simulink model "TEST_IPM_2_0"  (R2019b)
settings: configuration reference "Configuration" (kept outside this file)
PreLoadFcn:
  | RTWConfigurationCB('preloadfcn', bdroot);
values from neighbouring files (symbols this model uses):
  MParamFbase = 200.0    [TEST_IPM_LIB.sldd]
  MParamIbase = 360.0    [TEST_IPM_LIB.sldd]
  MParamLd = 0.002    [TEST_IPM_LIB.sldd]
  MParamLq = 0.002    [TEST_IPM_LIB.sldd]
  MParamRs = 1.15    [TEST_IPM_LIB.sldd]
  PWM_TPBRD_HALF = 5000.0    [TEST_IPM_LIB.sldd]
  Ts_10kHz = 0.0001    [TEST_IPM_LIB.sldd]
  Ts_1kHz = 0.001    [TEST_IPM_LIB.sldd]
undefined symbols (not defined in the file or in its folder): Down, GPTRIP1SEL, GPTRIP2SEL, TZ1, TZ2, Up
libraries: c280xlib x66, c2837xDlib x18, c2802xlib x10, powerlib_meascontrol x9, dsparch4 x4, c2000lib x1, c2806xlib x1, idelinklib_common x1
(part 3 of 6)

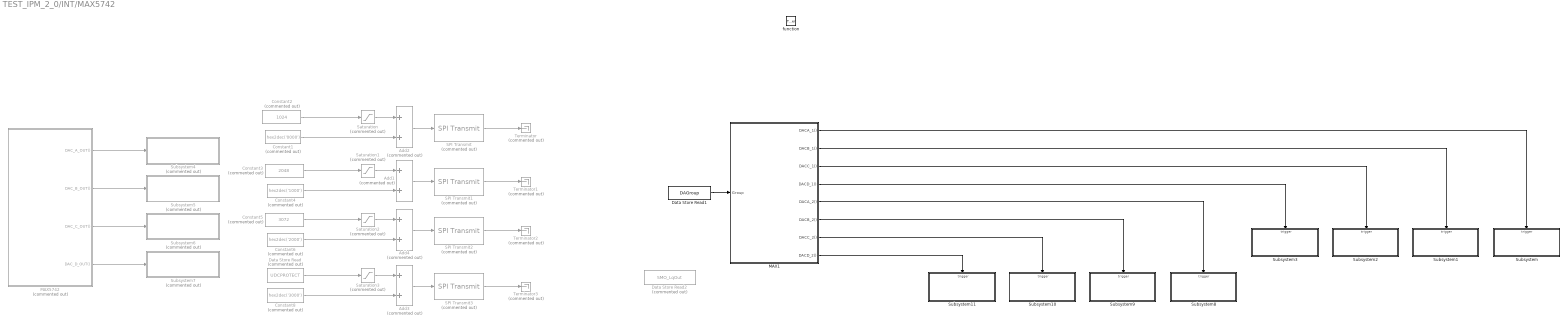
== system TEST_IPM_2_0/INT/MAX5742 ==
  function : TriggerPort  TriggerType=function-call  VariantControl=Variant
  Add{1..4} (4 alike) : Sum  Commented=on
  Constant1 : Constant  Commented=on  Value=hex2dec('0000')  OutDataTypeStr=uint16  SampleTime=-1
  Constant2 : Constant  Priority=102  Commented=on  Value=1024  OutDataTypeStr=Inherit: Inherit via back propagation  SampleTime=-1
  Constant3 : Constant  Priority=107  Commented=on  Value=2048  OutDataTypeStr=Inherit: Inherit via back propagation  SampleTime=-1
  Constant4 : Constant  Commented=on  Value=hex2dec('1000')  OutDataTypeStr=uint16  SampleTime=-1
  Constant5 : Constant  Priority=112  Commented=on  Value=3072  OutDataTypeStr=Inherit: Inherit via back propagation  SampleTime=-1
  Constant6 : Constant  Commented=on  Value=hex2dec('2000')  OutDataTypeStr=uint16  SampleTime=-1
  Constant8 : Constant  Commented=on  Value=hex2dec('3000')  OutDataTypeStr=uint16  SampleTime=-1
  Data Store Read : DataStoreRead  Commented=on  DataStoreName=UDCPROTECT
  Data Store Read1 : DataStoreRead  DataStoreName=DAGroup
  Data Store Read2 : DataStoreRead  Commented=on  DataStoreName=SMO_LqOut
  MAX1 : MATLAB Function  TreatAsAtomicUnit=on
  MAX5742 : Stateflow chart  Commented=on  BlockKeywords=__PRM__SERIALIZED__DATA__:Stateflow Chart,Stateflow Diagram  TreatAsAtomicUnit=on
  SPI Transmit : c280xlib/SPI Transmit  Commented=on  SPISelect=SPI_B  ClockPolarity=Falling_edge  ClockPhase=No_delay  SPIModule=uint32(0)  Mode=Master  BusSpeed=uint32(1000000)  FirstBitToTransfer=Most significant bit (MSB)  ClockMode=0  BlockFunction=Write  EnableRegisterAddress=on  RegisterAddress=0  OutputDataType=int8  OutputDataLength=1  BlockingMode=off  DataBits=16  UseCustomSSPin=Provided by the SPI peripheral  ActiveLowSSPin=Active low  Pin=0
      settings: SourceProductName=Embedded Coder Support Package for Texas Instruments C2000 Processors  SourceProductBaseCode=TIC2000
  SPI Transmit1 : c280xlib/SPI Transmit  Commented=on  SPISelect=SPI_B  ClockPolarity=Rising_edge  ClockPhase=No_delay  SPIModule=uint32(0)  Mode=Master  BusSpeed=uint32(1000000)  FirstBitToTransfer=Most significant bit (MSB)  ClockMode=0  BlockFunction=Write  EnableRegisterAddress=on  RegisterAddress=0  OutputDataType=int8  OutputDataLength=1  BlockingMode=off  DataBits=16  UseCustomSSPin=Provided by the SPI peripheral  ActiveLowSSPin=Active low  Pin=0
      settings: SourceProductName=Embedded Coder Support Package for Texas Instruments C2000 Processors  SourceProductBaseCode=TIC2000
  SPI Transmit2 : c280xlib/SPI Transmit  Commented=on  SPISelect=SPI_B  ClockPolarity=Rising_edge  ClockPhase=No_delay  SPIModule=uint32(0)  Mode=Master  BusSpeed=uint32(1000000)  FirstBitToTransfer=Most significant bit (MSB)  ClockMode=0  BlockFunction=Write  EnableRegisterAddress=on  RegisterAddress=0  OutputDataType=int8  OutputDataLength=1  BlockingMode=off  DataBits=16  UseCustomSSPin=Provided by the SPI peripheral  ActiveLowSSPin=Active low  Pin=0
      settings: SourceProductName=Embedded Coder Support Package for Texas Instruments C2000 Processors  SourceProductBaseCode=TIC2000
  SPI Transmit3 : c280xlib/SPI Transmit  Commented=on  SPISelect=SPI_B  ClockPolarity=Rising_edge  ClockPhase=No_delay  SPIModule=uint32(0)  Mode=Master  BusSpeed=uint32(1000000)  FirstBitToTransfer=Most significant bit (MSB)  ClockMode=0  BlockFunction=Write  EnableRegisterAddress=on  RegisterAddress=0  OutputDataType=int8  OutputDataLength=1  BlockingMode=off  DataBits=16  UseCustomSSPin=Provided by the SPI peripheral  ActiveLowSSPin=Active low  Pin=0
      settings: SourceProductName=Embedded Coder Support Package for Texas Instruments C2000 Processors  SourceProductBaseCode=TIC2000
  Saturation{,1..3} (4 alike) : Saturate  Commented=on  UpperLimit=4095  LowerLimit=0  OutDataTypeStr=uint16
  Subsystem : Subsystem
  Subsystem1 : Subsystem
  Subsystem10 : Subsystem
  Subsystem11 : Subsystem
  Subsystem2 : Subsystem
  Subsystem3 : Subsystem
  Subsystem4 : Subsystem  Commented=on
  Subsystem5 : Subsystem  Commented=on
  Subsystem6 : Subsystem  Commented=on
  Subsystem7 : Subsystem  Commented=on
  Subsystem8 : Subsystem
  Subsystem9 : Subsystem
  Terminator{,1..3} (4 alike) : Terminator  Commented=on
  wires:
  MAX1/4(DACD_1()) -> Subsystem3/Trigger
  MAX1/3(DACC_1()) -> Subsystem2/Trigger
  MAX1/2(DACB_1()) -> Subsystem1/Trigger
  MAX1/1(DACA_1()) -> Subsystem/Trigger
  SPI Transmit/1 -> Terminator/1
  Add2/1 -> SPI Transmit/1
  Saturation/1 -> Add2/1
  Constant2/1 -> Saturation/1
  Constant1/1 -> Add2/2
  SPI Transmit1/1 -> Terminator1/1
  Constant4/1 -> Add1/2
  Add1/1 -> SPI Transmit1/1
  Saturation1/1 -> Add1/1
  Constant3/1 -> Saturation1/1
  Constant5/1 -> Saturation2/1
  Constant6/1 -> Add4/2
  Add4/1 -> SPI Transmit2/1
  Saturation2/1 -> Add4/1
  SPI Transmit2/1 -> Terminator2/1
  Saturation3/1 -> Add3/1
  Add3/1 -> SPI Transmit3/1
  SPI Transmit3/1 -> Terminator3/1
  Constant8/1 -> Add3/2
  Data Store Read/1 -> Saturation3/1
  MAX5742/1(DAC_A_OUT()) -> Subsystem4/Trigger
  MAX5742/2(DAC_B_OUT()) -> Subsystem5/Trigger
  MAX5742/3(DAC_C_OUT()) -> Subsystem6/Trigger
  MAX5742/4(DAC_D_OUT()) -> Subsystem7/Trigger
  MAX1/5(DACA_2()) -> Subsystem8/Trigger
  MAX1/6(DACB_2()) -> Subsystem9/Trigger
  MAX1/7(DACC_2()) -> Subsystem10/Trigger
  MAX1/8(DACD_2()) -> Subsystem11/Trigger
  Data Store Read1/1 -> MAX1/1(Group)

== system TEST_IPM_2_0/INT/Motor Control ==
  function : TriggerPort  TriggerType=function-call  VariantControl=Variant
  Adjusting Mode : Subsystem  TreatAsAtomicUnit=on
  Clark Transformation : Subsystem
  Current_PI : Subsystem  TreatAsAtomicUnit=on
      settings: RTWSystemCode=Inline
  Data Store Read : DataStoreRead  DataStoreName=U_Current
  Data Store Read1 : DataStoreRead  DataStoreName=ControlAng
  Data Store Read2 : DataStoreRead  DataStoreName=ControlMode
  Data Store Read5 : DataStoreRead  DataStoreName=V_Current
  Data Store Read6 : DataStoreRead  DataStoreName=W_Current
  Data Store Write : DataStoreWrite  DataStoreName=COMPARE_A
  Data Store Write1 : DataStoreWrite  DataStoreName=COMPARE_B
  Data Store Write2 : DataStoreWrite  DataStoreName=COMPARE_C
  Data Store Write3 : DataStoreWrite  DataStoreName=Beta_Current
  Data Store Write4 : DataStoreWrite  DataStoreName=Alpha_Current
  Demux : Demux  Outputs=3
  Error : Subsystem  TreatAsAtomicUnit=on
  IF : Subsystem  TreatAsAtomicUnit=on
  Park Transformation : Subsystem
  SVPWM : Subsystem  TreatAsAtomicUnit=on
      settings: RTWSystemCode=Inline
  SpeedMode : Subsystem  TreatAsAtomicUnit=on
  "Stop " : Subsystem  TreatAsAtomicUnit=on
  Switch Case : SwitchCase  CaseConditions={0,1,2,3,4,5}
  TorqueMode : Subsystem  TreatAsAtomicUnit=on
  VF : Subsystem  TreatAsAtomicUnit=on
  wires:
  Data Store Read2/1 -> Switch Case/1
  Switch Case/1 -> Adjusting Mode/Action
  Switch Case/6 -> "Stop "/Action
  Switch Case/7 -> Error/Action
  Switch Case/2 -> VF/Action
  Switch Case/3 -> IF/Action
  Switch Case/4 -> TorqueMode/Action
  Switch Case/5 -> SpeedMode/Action
  Clark Transformation/2(Beta) -> Data Store Write3/1, Park Transformation/2(Beta)
  Clark Transformation/1(Alpha) -> Data Store Write4/1, Park Transformation/1(Alpha)
  Data Store Read1/1 -> SVPWM/3(Angle), Park Transformation/3(theta)
  Data Store Read/1 -> Clark Transformation/1(U)
  Data Store Read5/1 -> Clark Transformation/2(V)
  Data Store Read6/1 -> Clark Transformation/3(W)
  Park Transformation/1(D) -> Current_PI/1(Id_FeedBack)
  Park Transformation/2(Q) -> Current_PI/2(Iq_FeedBack)
  Current_PI/1(Ud_Reference) -> SVPWM/1(Ud_Reference)
  Current_PI/2(Uq_Reference) -> SVPWM/2(Uq_Reference)
  SVPWM/1(COMPARE) -> Demux/1
  Demux/1 -> Data Store Write/1
  Demux/2 -> Data Store Write1/1
  Demux/3 -> Data Store Write2/1

== system TEST_IPM_2_0/INT/Read Rotor Position ==
  function : TriggerPort  TriggerType=function-call  VariantControl=Variant
  Add : Sum  Inputs=+-  OutDataTypeStr=int16
  Constant1 : Constant  Value=10000  OutDataTypeStr=int16  SampleTime=-1
  Constant2 : Constant  Value=2*pi  OutDataTypeStr=single  SampleTime=-1
  Data Store Read : DataStoreRead  Priority=3  Commented=on  DataStoreName=SPIC_Tx
  Data Store Read1 : DataStoreRead  Priority=5  Commented=on  DataStoreName=SPIC_Tx
  Data Store Read2 : DataStoreRead  DataStoreName=QEP_OFFSET
  Data Store Read3 : DataStoreRead  Commented=on  DataStoreName=ResloverMid
  Data Store Write : DataStoreWrite  Commented=on  DataStoreName=ResloverAng
  Data Store Write1 : DataStoreWrite  Commented=on  DataStoreName=SPIC_Rx
  Data Store Write2 : DataStoreWrite  Commented=on  DataStoreName=N_FBK
  Data Store Write3 : DataStoreWrite  Commented=on  DataStoreName=ResloverFaultRead
  Data Store Write4 : DataStoreWrite  DataStoreName=QEP_RAW
  Data Store Write5 : DataStoreWrite  DataStoreName=ResloverAng
  Data Store Write6 : DataStoreWrite  DataStoreName=QEP_ANGLE
  Data Store Write7 : DataStoreWrite  DataStoreName=N_FBK
  Digital Output1 : c2837xDlib/Digital Output  Commented=on  GPIO_Number=GPIO48~GPIO55  GPIO_Bit0=off  GPIO_BIT0_Toggle=off  GPIO_Bit1=off  GPIO_BIT1_Toggle=off  GPIO_Bit2=off  GPIO_BIT2_Toggle=off  GPIO_Bit3=off  GPIO_BIT3_Toggle=off  GPIO_Bit4=off  GPIO_BIT4_Toggle=off  GPIO_Bit5=on  GPIO_BIT5_Toggle=off  GPIO_Bit6=off  GPIO_BIT6_Toggle=off  GPIO_Bit7=off  GPIO_BIT7_Toggle=off
      settings: SourceProductName=Embedded Coder Support Package for Texas Instruments C2000 Processors  SourceProductBaseCode=TIC2000
  Digital Output2 : c2837xDlib/Digital Output  Commented=on  GPIO_Number=GPIO48~GPIO55  GPIO_Bit0=off  GPIO_BIT0_Toggle=off  GPIO_Bit1=off  GPIO_BIT1_Toggle=off  GPIO_Bit2=off  GPIO_BIT2_Toggle=off  GPIO_Bit3=off  GPIO_BIT3_Toggle=off  GPIO_Bit4=off  GPIO_BIT4_Toggle=off  GPIO_Bit5=off  GPIO_BIT5_Toggle=off  GPIO_Bit6=on  GPIO_BIT6_Toggle=off  GPIO_Bit7=off  GPIO_BIT7_Toggle=off
      settings: SourceProductName=Embedded Coder Support Package for Texas Instruments C2000 Processors  SourceProductBaseCode=TIC2000
  Gain : Gain  Commented=on  Gain=2*pi
  Gain1 : Gain  Gain=5  OutDataTypeStr=single
  Gain2 : Gain  Gain=2*pi/10000  OutDataTypeStr=single
  MATLAB Function : MATLAB Function  Commented=on  TreatAsAtomicUnit=on
  MATLAB Function1 : MATLAB Function  TreatAsAtomicUnit=on
  Mod : Math  Operator=mod  SignedPower=off  OutputSignalType=real  SaturateOnIntegerOverflow=on
  Mod1 : Math  Operator=mod  SignedPower=off  OutputSignalType=real  SaturateOnIntegerOverflow=on
  "RAW_DATA2Angle " : MATLAB Function  Commented=on  TreatAsAtomicUnit=on
  ResloverWR1 : Constant  Priority=6  Commented=on  OutDataTypeStr=Inherit: Inherit via back propagation  SampleTime=-1
  ResloverWR2 : Constant  Priority=6  Commented=on  OutDataTypeStr=Inherit: Inherit via back propagation  SampleTime=-1
  SPI Master Transfer : c280xlib/SPI Master Transfer  Commented=on  SPISelect=SPI_C  ClockPolarity=Rising_edge  ClockPhase=No_delay  SPIModule=uint32(0)  Mode=Master  BusSpeed=uint32(1000000)  FirstBitToTransfer=Most significant bit (MSB)  ClockMode=0  BlockFunction=Transfer  EnableRegisterAddress=off  RegisterAddress=0  OutputDataType=int8  OutputDataLength=1  DataBits=16  UseCustomSSPin=Provided by the SPI peripheral  ActiveLowSSPin=Active low  Pin=1
      settings: SourceProductName=Embedded Coder Support Package for Texas Instruments C2000 Processors  SourceProductBaseCode=TIC2000
  SPI Master Transfer1 : c280xlib/SPI Master Transfer  Commented=on  SPISelect=SPI_C  ClockPolarity=Rising_edge  ClockPhase=No_delay  SPIModule=uint32(0)  Mode=Master  BusSpeed=uint32(1000000)  FirstBitToTransfer=Most significant bit (MSB)  ClockMode=0  BlockFunction=Transfer  EnableRegisterAddress=off  RegisterAddress=0  OutputDataType=int8  OutputDataLength=1  DataBits=8  UseCustomSSPin=Provided by the SPI peripheral  ActiveLowSSPin=Active low  Pin=1
      settings: SourceProductName=Embedded Coder Support Package for Texas Instruments C2000 Processors  SourceProductBaseCode=TIC2000
  SpeedCal : Subsystem  Commented=on  TreatAsAtomicUnit=on
  SpeedCal1 : Subsystem  TreatAsAtomicUnit=on
  eQEP : c280xlib/eQEP  useModule=eQEP2  pcInputmode=Quadrature-count  externalClockrate=2x resolution: Count the rising/falling edge  swapPolarityselection=Clockwise  qdfOutputport=off  qapPolarityselection=off  qbpPolarityselection=off  qipPolarityselection=off  qspPolarityselection=off  igatePolarityselection=off  sampleTime=-1  pcOutputport=on  pcMaximumvalue=10000  indexInitializationcheck=off  indexInitializationevent=Rising edge  strobeInitializationcheck=off  strobeInitializationevent=Rising edge  softwareInitializationcheck=off  softwareInitializationsource=Set to init value at start up  softwareInitializationmode=on  pcInitialvalue=2147483648  pcResetmode=Reset on an index event  ieloutputport=off  indexEventlatch=Rising edge  seloutputport=off  strobeEventlatch=Rising edge  pcefOutputport=off  enableEqepcapture=off  qctmrOutputport=off  qcprdOutputport=off  captureTimerprescaler=128  upEventprescaler=128  overflowErrorflag=off  directionErrorflag=off  captureTimerposition=On position counter read  unitTimerperiod=100000000  captureTimerlatch=off  capturePeriodlatch=off  positionCounterlatch=off  soenPolarityselection=off  spselPolarityselection=Index pin is used for sync output  compareValuesource=Specify via dialog  shadowMode=Load on QPOSCNT=0  compareValue=4294967295  syncOutputwidth=1  polaritySyncoutput=Active high  watchdogEnable=off  watchdogTimer=65535  outport1Datatype=auto  outport2Datatype=auto  outport3Datatype=auto  outport4Datatype=auto  outport5Datatype=auto  outport6Datatype=auto  outport7Datatype=auto  outport8Datatype=auto  outport9Datatype=auto  outport10Datatype=auto  outport11Datatype=auto  outport12Datatype=auto  eqepinterrupt_pce=off  eqepinterrupt_qpe=off  eqepinterrupt_qdc=off  eqepinterrupt_wto=off  eqepinterrupt_pcu=off  eqepinterrupt_pco=off  eqepinterrupt_pcr=off  eqepinterrupt_pcm=off  eqepinterrupt_sel=off  eqepinterrupt_iel=off  eqepinterrupt_uto=off  pheOutputport=off  watchdogOutputport=off  outport13Datatype=auto  outport14Datatype=auto
      settings: SourceProductName=Embedded Coder Support Package for Texas Instruments C2000 Processors  SourceProductBaseCode=TIC2000
  wires:
  Data Store Read/1 -> SPI Master Transfer/1
  SPI Master Transfer/1 -> Data Store Write1/1, "RAW_DATA2Angle "/1(Raw_Data)
  ResloverWR1/1 -> Digital Output1/1
  Data Store Read3/1 -> "RAW_DATA2Angle "/2(Mid_Position)
  "RAW_DATA2Angle "/1(Angle_out) -> Gain/1
  SpeedCal/1(Out1) -> Data Store Write2/1
  MATLAB Function/1(FunCall()) -> SpeedCal/Trigger
  Data Store Read1/1 -> SPI Master Transfer1/1
  SPI Master Transfer1/1 -> Data Store Write3/1
  ResloverWR2/1 -> Digital Output2/1
  Gain/1 -> SpeedCal/1(In1), Data Store Write/1
  eQEP/1 -> Data Store Write4/1, Add/1
  Data Store Read2/1 -> Add/2
  Add/1 -> Mod/1
  Mod/1 -> Gain2/1
  Constant1/1 -> Mod/2
  Gain2/1 -> Gain1/1, SpeedCal1/1(In1), Data Store Write6/1
  Mod1/1 -> Data Store Write5/1
  Gain1/1 -> Mod1/1
  Constant2/1 -> Mod1/2
  MATLAB Function1/1(FunCall()) -> SpeedCal1/Trigger
  SpeedCal1/1(Out1) -> Data Store Write7/1

== system TEST_IPM_2_0/INT/ePWM ==
  function : TriggerPort  TriggerType=function-call  VariantControl=Variant
  Constant2 : Constant  Value=[0 0]  OutDataTypeStr=uint16  SampleTime=-1
  Constant3 : Constant  Value=[1 2]  OutDataTypeStr=uint16  SampleTime=-1
  Data Store Read1 : DataStoreRead  DataStoreName=STOP
  Data Store Read3 : DataStoreRead  DataStoreName=COMPARE_A
  Data Store Read4 : DataStoreRead  DataStoreName=COMPARE_B
  Data Store Read7 : DataStoreRead  DataStoreName=COMPARE_C
  Demux : Demux  Outputs=2
  If : If  IfExpression=u1 == 1
  If Action Subsystem : Subsystem  TreatAsAtomicUnit=on
  Switch : Switch  Criteria=u2 ~= 0
  ePWM : c2802xlib/ePWM  useModule=ePWM1  ePWMxLINKTBPRD=Not Linked  periodUnits=Clock cycles  timerSource=Specify via dialog  timerPeriod_clk=PWM_TPBRD  timerPeriod_sec=Tsw  tbshadow=Counter equals to zero  countingMode=Up-Down  phaseActiveEnable=Disable  phaseDirection=Count down after sync  phaseActive=0  synchronizationEnable=off  dcaevt1Sync=off  dcbevt1Sync=off  synchronizationOption=Counter equals to zero (CTR=Zero)  clockPrescale=1  HSclockPrescale=1  enswap=off  ePWMxAStatus=on  ePWMxAactionLogic1=Do nothing  ePWMxAactionLogic2=Do nothing  ePWMxAactionLogic3=Clear  ePWMxAactionLogic4=Set  ePWMxAactionLogic5=Do nothing  ePWMxAactionLogic6=Do nothing  ePWMxALoadMode=Load on counter equals to zero (CTR=Zero)  ePWMxACSFenable=on  ePWMxACSFvalue=Forcing disable  ePWMxASFreload=Immediate  ePWMxBStatus=on  ePWMxBactionLogic1=Do nothing  ePWMxBactionLogic2=Do nothing  ePWMxBactionLogic3=Clear  ePWMxBactionLogic4=Set  ePWMxBactionLogic5=Do nothing  ePWMxBactionLogic6=Do nothing  ePWMxBLoadMode=Load on counter equals to zero (CTR=Zero)  ePWMxBCSFenable=on  ePWMxBCSFvalue=Forcing disable  ePWMxBSFreload=Immediate  ePWNxBOutWay=off  ePWMxLINKCMPA=Not Linked  CMPAUnits=Clock cycles  CMPASource=Input port  CMPAValue_per=50  CMPAValue_clk=PWM_TPBRD_HALF  enCMPAshadow=Counter equals to zero  ePWMxLINKCMPB=Not Linked  CMPBUnits=Percentages  CMPBSource=Specify via dialog  CMPBValue_per=50  CMPBValue_clk=32000  enCMPBshadow=Counter equals to zero  ePWMxLINKCMPC=Not Linked  CMPCUnits=Clock cycles  CMPCSource=Specify via dialog  CMPCValue_per=50  CMPCValue_clk=32000  enCMPCshadow=Counter equals to zero  ePWMxLINKCMPD=Not Linked  CMPDUnits=Clock cycles  CMPDSource=Specify via dialog  CMPDValue_per=50  CMPDValue_clk=32000  enCMPDshadow=Counter equals to zero  enableDBePWMxA=on  enableDBePWMxB=on  enhalfcycle=off  DBpolarity=Active high complementary (AHC)  DBedgeDelay=Positive  DBSource_ePWMxA=ePWMxA  DBSource_ePWMxB=ePWMxB  DBperiodSource=Specify via dialog  REDperiod=PWM_TDEAD  FEDperiod=PWM_TDEAD  adcstartModuleA=on  adcrequestEventA=First event  adcstartEventA=Digital Compare Module A Event 1 start of conversion (DCAEVT1.soc)  adcstartEventA_type2=Counter equals to zero (CTR=Zero)  adcstartModuleB=off  adcrequestEventB=First event  adcstartEventB=Counter equals to zero (CTR=Zero)  adcstartEventB_type2=Counter equals to zero (CTR=Zero)  intEn=off  intPrd=First event  intSel=Counter equals to zero (CTR=Zero)  intSel_type2=Counter equals to period (CTR=PRD)  hrpe=off  enHRPWM=off  HRPWM_LoadMode=Counter equals to period (CTR=PRD)  HRPWM_CTLMode=Duty or Period control mode  HRPWM_EDGMode=Both edge  hrpeb=off  enHRPWMB=off  HRPWM_LoadModeB=Counter equals to zero (CTR=ZERO)  HRPWM_CTLModeB=Duty or Period control mode  HRPWM_EDGModeB=Both edge  enSFO=on  enautoconv=on  chopperEnable=off  chopperFrequency=1  chopperFirstwidth=1  chopperDuty=12.5%  tripZonesource=Specify via dialog  tzselOSHT1=off  tzselOSHT2=off  tzselOSHT3=off  tzselOSHDCAEV1=off  tzselOSHDCBEV1=off  tzselCBC1=off  tzselCBC2=off  tzselCBC3=off  tzselCBCDCAEV2=off  tzselCBCDCBEV2=off  tzselOSHT4=off  tzselOSHT5=off  tzselOSHT6=off  tzselCBC4=off  tzselCBC5=off  tzselCBC6=off  enTzOstIntr=on  enTzCbcIntr=off  enTzDCAEVT1Intr=off  enTzDCAEVT2Intr=off  enTzDCBEVT1Intr=off  enTzDCBEVT2Intr=off  ePWMxAforced=Low  ePWMxBforced=Low  DCAEVT1forced=No action  DCBEVT1forced=No action  DCAEVT2forced=No action  DCBEVT2forced=No action  dcah=Trip Zone 1 input (TZ1)  dcal=Trip Zone 2 input (TZ2)  dcbh=Trip Zone 1 input (TZ1)  dcbl=Trip Zone 2 input (TZ2)  dcah_type2=GPTRIP1SEL/(TZ1)  dcal_type2=GPTRIP2SEL/(TZ2)  dcbh_type2=GPTRIP1SEL/(TZ1)  dcbl_type2=GPTRIP2SEL/(TZ2)  gendcaevt1=Event disabled  gendcaevt2=Event disabled  gendcbevt1=Event disabled  gendcbevt2=Event disabled  dcaevt1src=DCAEVT1 with sync  dcaevt2src=DCAEVT2 with sync  dcbevt1src=DCBEVT1 with sync  dcbevt2src=DCBEVT2 with sync  pulsesel=Counter equals to zero (CTR=Zero)  blankinv=off  blankoffset=0  blankwidth=0  evsrcsel=Filtered version of DCAEVT1 (DCAEVT1FILT)  encape=off  PwmType=C2000_Type4
      settings: SourceProductName=Embedded Coder Support Package for Texas Instruments C2000 Processors
  ePWM1 : c2802xlib/ePWM  useModule=ePWM2  ePWMxLINKTBPRD=Not Linked  periodUnits=Clock cycles  timerSource=Specify via dialog  timerPeriod_clk=PWM_TPBRD  timerPeriod_sec=Tsw  tbshadow=Counter equals to zero  countingMode=Up-Down  phaseActiveEnable=Set counter to phase value specified via dialog  phaseDirection=Count down after sync  phaseActive=0  synchronizationEnable=off  dcaevt1Sync=off  dcbevt1Sync=off  synchronizationOption=Disable  clockPrescale=1  HSclockPrescale=1  enswap=off  ePWMxAStatus=on  ePWMxAactionLogic1=Do nothing  ePWMxAactionLogic2=Do nothing  ePWMxAactionLogic3=Clear  ePWMxAactionLogic4=Set  ePWMxAactionLogic5=Do nothing  ePWMxAactionLogic6=Do nothing  ePWMxALoadMode=Load on counter equals to zero (CTR=Zero)  ePWMxACSFenable=on  ePWMxACSFvalue=Forcing disable  ePWMxASFreload=Immediate  ePWMxBStatus=on  ePWMxBactionLogic1=Do nothing  ePWMxBactionLogic2=Do nothing  ePWMxBactionLogic3=Clear  ePWMxBactionLogic4=Set  ePWMxBactionLogic5=Do nothing  ePWMxBactionLogic6=Do nothing  ePWMxBLoadMode=Load on counter equals to zero (CTR=Zero)  ePWMxBCSFenable=on  ePWMxBCSFvalue=Forcing disable  ePWMxBSFreload=Immediate  ePWNxBOutWay=off  ePWMxLINKCMPA=Not Linked  CMPAUnits=Clock cycles  CMPASource=Input port  CMPAValue_per=50  CMPAValue_clk=PWM_TPBRD_HALF  enCMPAshadow=Counter equals to zero  ePWMxLINKCMPB=Not Linked  CMPBUnits=Percentages  CMPBSource=Specify via dialog  CMPBValue_per=50  CMPBValue_clk=32000  enCMPBshadow=Counter equals to zero  ePWMxLINKCMPC=Not Linked  CMPCUnits=Clock cycles  CMPCSource=Specify via dialog  CMPCValue_per=50  CMPCValue_clk=32000  enCMPCshadow=Counter equals to zero  ePWMxLINKCMPD=Not Linked  CMPDUnits=Clock cycles  CMPDSource=Specify via dialog  CMPDValue_per=50  CMPDValue_clk=32000  enCMPDshadow=Counter equals to zero  enableDBePWMxA=on  enableDBePWMxB=on  enhalfcycle=off  DBpolarity=Active high complementary (AHC)  DBedgeDelay=Positive  DBSource_ePWMxA=ePWMxA  DBSource_ePWMxB=ePWMxB  DBperiodSource=Specify via dialog  REDperiod=PWM_TDEAD  FEDperiod=PWM_TDEAD  adcstartModuleA=off  adcrequestEventA=First event  adcstartEventA=Digital Compare Module A Event 1 start of conversion (DCAEVT1.soc)  adcstartEventA_type2=Counter equals to period (CTR=PRD)  adcstartModuleB=off  adcrequestEventB=First event  adcstartEventB=Counter equals to zero (CTR=Zero)  adcstartEventB_type2=Counter equals to zero (CTR=Zero)  intEn=off  intPrd=First event  intSel=Counter equals to zero (CTR=Zero)  intSel_type2=Counter equals to period (CTR=PRD)  hrpe=off  enHRPWM=off  HRPWM_LoadMode=Counter equals to period (CTR=PRD)  HRPWM_CTLMode=Duty or Period control mode  HRPWM_EDGMode=Both edge  hrpeb=off  enHRPWMB=off  HRPWM_LoadModeB=Counter equals to zero (CTR=ZERO)  HRPWM_CTLModeB=Duty or Period control mode  HRPWM_EDGModeB=Both edge  enSFO=on  enautoconv=on  chopperEnable=off  chopperFrequency=1  chopperFirstwidth=1  chopperDuty=12.5%  tripZonesource=Specify via dialog  tzselOSHT1=off  tzselOSHT2=off  tzselOSHT3=off  tzselOSHDCAEV1=off  tzselOSHDCBEV1=off  tzselCBC1=off  tzselCBC2=off  tzselCBC3=off  tzselCBCDCAEV2=off  tzselCBCDCBEV2=off  tzselOSHT4=off  tzselOSHT5=off  tzselOSHT6=off  tzselCBC4=off  tzselCBC5=off  tzselCBC6=off  enTzOstIntr=on  enTzCbcIntr=off  enTzDCAEVT1Intr=off  enTzDCAEVT2Intr=off  enTzDCBEVT1Intr=off  enTzDCBEVT2Intr=off  ePWMxAforced=Low  ePWMxBforced=Low  DCAEVT1forced=No action  DCBEVT1forced=No action  DCAEVT2forced=No action  DCBEVT2forced=No action  dcah=Trip Zone 1 input (TZ1)  dcal=Trip Zone 2 input (TZ2)  dcbh=Trip Zone 1 input (TZ1)  dcbl=Trip Zone 2 input (TZ2)  dcah_type2=GPTRIP1SEL/(TZ1)  dcal_type2=GPTRIP2SEL/(TZ2)  dcbh_type2=GPTRIP1SEL/(TZ1)  dcbl_type2=GPTRIP2SEL/(TZ2)  gendcaevt1=Event disabled  gendcaevt2=Event disabled  gendcbevt1=Event disabled  gendcbevt2=Event disabled  dcaevt1src=DCAEVT1 with sync  dcaevt2src=DCAEVT2 with sync  dcbevt1src=DCBEVT1 with sync  dcbevt2src=DCBEVT2 with sync  pulsesel=Counter equals to zero (CTR=Zero)  blankinv=off  blankoffset=0  blankwidth=0  evsrcsel=Filtered version of DCAEVT1 (DCAEVT1FILT)  encape=off  PwmType=C2000_Type4
      settings: SourceProductName=Embedded Coder Support Package for Texas Instruments C2000 Processors
  ePWM2 : c2802xlib/ePWM  useModule=ePWM3  ePWMxLINKTBPRD=Not Linked  periodUnits=Clock cycles  timerSource=Specify via dialog  timerPeriod_clk=PWM_TPBRD  timerPeriod_sec=Tsw  tbshadow=Counter equals to zero  countingMode=Up-Down  phaseActiveEnable=Set counter to phase value specified via dialog  phaseDirection=Count down after sync  phaseActive=0  synchronizationEnable=off  dcaevt1Sync=off  dcbevt1Sync=off  synchronizationOption=Disable  clockPrescale=1  HSclockPrescale=1  enswap=off  ePWMxAStatus=on  ePWMxAactionLogic1=Do nothing  ePWMxAactionLogic2=Do nothing  ePWMxAactionLogic3=Clear  ePWMxAactionLogic4=Set  ePWMxAactionLogic5=Do nothing  ePWMxAactionLogic6=Do nothing  ePWMxALoadMode=Load on counter equals to zero (CTR=Zero)  ePWMxACSFenable=on  ePWMxACSFvalue=Forcing disable  ePWMxASFreload=Immediate  ePWMxBStatus=on  ePWMxBactionLogic1=Do nothing  ePWMxBactionLogic2=Do nothing  ePWMxBactionLogic3=Clear  ePWMxBactionLogic4=Set  ePWMxBactionLogic5=Do nothing  ePWMxBactionLogic6=Do nothing  ePWMxBLoadMode=Load on counter equals to zero (CTR=Zero)  ePWMxBCSFenable=on  ePWMxBCSFvalue=Forcing disable  ePWMxBSFreload=Immediate  ePWNxBOutWay=off  ePWMxLINKCMPA=Not Linked  CMPAUnits=Clock cycles  CMPASource=Input port  CMPAValue_per=50  CMPAValue_clk=PWM_TPBRD_HALF  enCMPAshadow=Counter equals to zero  ePWMxLINKCMPB=Not Linked  CMPBUnits=Percentages  CMPBSource=Specify via dialog  CMPBValue_per=50  CMPBValue_clk=32000  enCMPBshadow=Counter equals to zero  ePWMxLINKCMPC=Not Linked  CMPCUnits=Clock cycles  CMPCSource=Specify via dialog  CMPCValue_per=50  CMPCValue_clk=32000  enCMPCshadow=Counter equals to zero  ePWMxLINKCMPD=Not Linked  CMPDUnits=Clock cycles  CMPDSource=Specify via dialog  CMPDValue_per=50  CMPDValue_clk=32000  enCMPDshadow=Counter equals to zero  enableDBePWMxA=on  enableDBePWMxB=on  enhalfcycle=off  DBpolarity=Active high complementary (AHC)  DBedgeDelay=Positive  DBSource_ePWMxA=ePWMxA  DBSource_ePWMxB=ePWMxB  DBperiodSource=Specify via dialog  REDperiod=PWM_TDEAD  FEDperiod=PWM_TDEAD  adcstartModuleA=off  adcrequestEventA=First event  adcstartEventA=Digital Compare Module A Event 1 start of conversion (DCAEVT1.soc)  adcstartEventA_type2=Counter equals to zero (CTR=Zero)  adcstartModuleB=off  adcrequestEventB=First event  adcstartEventB=Counter equals to zero (CTR=Zero)  adcstartEventB_type2=Counter equals to zero (CTR=Zero)  intEn=off  intPrd=First event  intSel=Counter equals to zero (CTR=Zero)  intSel_type2=Counter equals to period (CTR=PRD)  hrpe=off  enHRPWM=off  HRPWM_LoadMode=Counter equals to period (CTR=PRD)  HRPWM_CTLMode=Duty or Period control mode  HRPWM_EDGMode=Both edge  hrpeb=off  enHRPWMB=off  HRPWM_LoadModeB=Counter equals to zero (CTR=ZERO)  HRPWM_CTLModeB=Duty or Period control mode  HRPWM_EDGModeB=Both edge  enSFO=on  enautoconv=on  chopperEnable=off  chopperFrequency=1  chopperFirstwidth=1  chopperDuty=12.5%  tripZonesource=Specify via dialog  tzselOSHT1=off  tzselOSHT2=off  tzselOSHT3=off  tzselOSHDCAEV1=off  tzselOSHDCBEV1=off  tzselCBC1=off  tzselCBC2=off  tzselCBC3=off  tzselCBCDCAEV2=off  tzselCBCDCBEV2=off  tzselOSHT4=off  tzselOSHT5=off  tzselOSHT6=off  tzselCBC4=off  tzselCBC5=off  tzselCBC6=off  enTzOstIntr=on  enTzCbcIntr=off  enTzDCAEVT1Intr=off  enTzDCAEVT2Intr=off  enTzDCBEVT1Intr=off  enTzDCBEVT2Intr=off  ePWMxAforced=Low  ePWMxBforced=Low  DCAEVT1forced=No action  DCBEVT1forced=No action  DCAEVT2forced=No action  DCBEVT2forced=No action  dcah=Trip Zone 1 input (TZ1)  dcal=Trip Zone 2 input (TZ2)  dcbh=Trip Zone 1 input (TZ1)  dcbl=Trip Zone 2 input (TZ2)  dcah_type2=GPTRIP1SEL/(TZ1)  dcal_type2=GPTRIP2SEL/(TZ2)  dcbh_type2=GPTRIP1SEL/(TZ1)  dcbl_type2=GPTRIP2SEL/(TZ2)  gendcaevt1=Event disabled  gendcaevt2=Event disabled  gendcbevt1=Event disabled  gendcbevt2=Event disabled  dcaevt1src=DCAEVT1 with sync  dcaevt2src=DCAEVT2 with sync  dcbevt1src=DCBEVT1 with sync  dcbevt2src=DCBEVT2 with sync  pulsesel=Counter equals to zero (CTR=Zero)  blankinv=off  blankoffset=0  blankwidth=0  evsrcsel=Filtered version of DCAEVT1 (DCAEVT1FILT)  encape=off  PwmType=C2000_Type4
      settings: SourceProductName=Embedded Coder Support Package for Texas Instruments C2000 Processors
  wires:
  Constant3/1 -> Switch/1
  Constant2/1 -> Switch/3
  Demux/2 -> ePWM1/3, ePWM/3, ePWM2/3
  Data Store Read1/1 -> If/1, Switch/2
  Switch/1 -> Demux/1
  Demux/1 -> ePWM2/2, ePWM1/2, ePWM/2
  Data Store Read7/1 -> ePWM2/1
  Data Store Read3/1 -> ePWM/1
  Data Store Read4/1 -> ePWM1/1
  If/1 -> If Action Subsystem/Action

== system TEST_IPM_2_0/SpeedREF/First Order Filter  ==
  input : Inport
  Add : Sum  Inputs=+-
  Add3 : Sum  AccumDataTypeStr=single
  Constant : Constant  OutDataTypeStr=single  SampleTime=-1
  Data Store Read1 : DataStoreRead  DataStoreName=N_Filter
  Data Store Read2 : DataStoreRead  DataStoreName=N_Filter
  Gain : Gain  Gain=2*pi*Ts_1kHz
  Gain1 : Gain  Gain=2*pi*Ts_1kHz
  Product : Product
  Product1 : Product
  Unit Delay3 : UnitDelay  SampleTime=-1  HasFrameUpgradeWarning=on
  "output " : Outport
  wires:
  input/1 -> Product/1
  Product/1 -> Add3/1
  Product1/1 -> Unit Delay3/1
  Add3/1 -> Product1/1, "output "/1
  Unit Delay3/1 -> Add3/2
  Data Store Read2/1 -> Gain/1
  Gain/1 -> Product/2
  Data Store Read1/1 -> Gain1/1
  Add/1 -> Product1/2
  Gain1/1 -> Add/2
  Constant/1 -> Add/1

== system TEST_IPM_2_0/SpeedREF/Subsystem1 ==
  TargetValue : Inport
  Step : Inport  Port=2
  MATLAB Function : MATLAB Function  TreatAsAtomicUnit=on
  Unit Delay : UnitDelay  SampleTime=-1  HasFrameUpgradeWarning=on
  RampOutput : Outport
  wires:
  TargetValue/1 -> MATLAB Function/1(Target)
  MATLAB Function/1(Output) -> RampOutput/1, Unit Delay/1
  Step/1 -> MATLAB Function/2(Step)
  Unit Delay/1 -> MATLAB Function/3(LastOutput)

== system TEST_IPM_2_0/INT/AD2S1210 Init/Function-Call Subsystem ==
  function : TriggerPort  TriggerType=function-call  VariantControl=Variant
  Data Store Read : DataStoreRead  DataStoreName=ResloverRESET
  Digital Output : c2837xDlib/Digital Output  GPIO_Number=GPIO48~GPIO55  GPIO_Bit0=off  GPIO_BIT0_Toggle=off  GPIO_Bit1=off  GPIO_BIT1_Toggle=off  GPIO_Bit2=off  GPIO_BIT2_Toggle=off  GPIO_Bit3=off  GPIO_BIT3_Toggle=off  GPIO_Bit4=off  GPIO_BIT4_Toggle=off  GPIO_Bit5=off  GPIO_BIT5_Toggle=off  GPIO_Bit6=off  GPIO_BIT6_Toggle=off  GPIO_Bit7=on  GPIO_BIT7_Toggle=off
      settings: SourceProductName=Embedded Coder Support Package for Texas Instruments C2000 Processors  SourceProductBaseCode=TIC2000
  wires:
  Data Store Read/1 -> Digital Output/1

== system TEST_IPM_2_0/INT/AD2S1210 Init/Function-Call Subsystem1 ==
  function : TriggerPort  TriggerType=function-call  VariantControl=Variant
  Data Store Read : DataStoreRead  DataStoreName=ResloverWR
  Digital Output : c2837xDlib/Digital Output  GPIO_Number=GPIO48~GPIO55  GPIO_Bit0=off  GPIO_BIT0_Toggle=off  GPIO_Bit1=off  GPIO_BIT1_Toggle=off  GPIO_Bit2=off  GPIO_BIT2_Toggle=off  GPIO_Bit3=off  GPIO_BIT3_Toggle=off  GPIO_Bit4=off  GPIO_BIT4_Toggle=off  GPIO_Bit5=on  GPIO_BIT5_Toggle=off  GPIO_Bit6=off  GPIO_BIT6_Toggle=off  GPIO_Bit7=off  GPIO_BIT7_Toggle=off
      settings: SourceProductName=Embedded Coder Support Package for Texas Instruments C2000 Processors  SourceProductBaseCode=TIC2000
  wires:
  Data Store Read/1 -> Digital Output/1

== system TEST_IPM_2_0/INT/AD2S1210 Init/Function-Call Subsystem2 ==
  function : TriggerPort  TriggerType=function-call  VariantControl=Variant
  Data Store Read : DataStoreRead  Priority=1  DataStoreName=ResloverWR
  Data Store Read1 : DataStoreRead  Priority=4  DataStoreName=SPIC_Tx
  Data Store Write : DataStoreWrite  DataStoreName=SPIC_Rx
  Digital Output : c2837xDlib/Digital Output  GPIO_Number=GPIO48~GPIO55  GPIO_Bit0=off  GPIO_BIT0_Toggle=off  GPIO_Bit1=off  GPIO_BIT1_Toggle=off  GPIO_Bit2=off  GPIO_BIT2_Toggle=off  GPIO_Bit3=off  GPIO_BIT3_Toggle=off  GPIO_Bit4=off  GPIO_BIT4_Toggle=off  GPIO_Bit5=on  GPIO_BIT5_Toggle=off  GPIO_Bit6=off  GPIO_BIT6_Toggle=off  GPIO_Bit7=off  GPIO_BIT7_Toggle=off
      settings: SourceProductName=Embedded Coder Support Package for Texas Instruments C2000 Processors  SourceProductBaseCode=TIC2000
  S-Function1 : S-Function  Priority=3  Commented=on  FunctionName=User_Defined_Code  Parameters=code  SFunctionDeploymentMode=off  EnableBusSupport=off  mask{code=DELAY_US(1u);}
  SPI Master Transfer : c280xlib/SPI Master Transfer  SPISelect=SPI_C  ClockPolarity=Rising_edge  ClockPhase=No_delay  SPIModule=uint32(0)  Mode=Master  BusSpeed=uint32(1000000)  FirstBitToTransfer=Most significant bit (MSB)  ClockMode=0  BlockFunction=Transfer  EnableRegisterAddress=off  RegisterAddress=0  OutputDataType=int8  OutputDataLength=1  DataBits=16  UseCustomSSPin=Provided by the SPI peripheral  ActiveLowSSPin=Active low  Pin=1
      settings: SourceProductName=Embedded Coder Support Package for Texas Instruments C2000 Processors  SourceProductBaseCode=TIC2000
  wires:
  Data Store Read1/1 -> SPI Master Transfer/1
  SPI Master Transfer/1 -> Data Store Write/1
  Data Store Read/1 -> Digital Output/1

== system TEST_IPM_2_0/INT/AD2S1210 Init/Function-Call Subsystem3 ==
  function : TriggerPort  TriggerType=function-call  VariantControl=Variant
  Data Store Read : DataStoreRead  DataStoreName=ResloverA0
  Data Store Read1 : DataStoreRead  DataStoreName=ResloverA1
  Digital Output : c2837xDlib/Digital Output  GPIO_Number=GPIO56~GPIO63  GPIO_Bit0=off  GPIO_BIT0_Toggle=off  GPIO_Bit1=off  GPIO_BIT1_Toggle=off  GPIO_Bit2=on  GPIO_BIT2_Toggle=off  GPIO_Bit3=off  GPIO_BIT3_Toggle=off  GPIO_Bit4=off  GPIO_BIT4_Toggle=off  GPIO_Bit5=off  GPIO_BIT5_Toggle=off  GPIO_Bit6=off  GPIO_BIT6_Toggle=off  GPIO_Bit7=off  GPIO_BIT7_Toggle=off
      settings: SourceProductName=Embedded Coder Support Package for Texas Instruments C2000 Processors  SourceProductBaseCode=TIC2000
  Digital Output1 : c2837xDlib/Digital Output  GPIO_Number=GPIO56~GPIO63  GPIO_Bit0=off  GPIO_BIT0_Toggle=off  GPIO_Bit1=off  GPIO_BIT1_Toggle=off  GPIO_Bit2=off  GPIO_BIT2_Toggle=off  GPIO_Bit3=on  GPIO_BIT3_Toggle=off  GPIO_Bit4=off  GPIO_BIT4_Toggle=off  GPIO_Bit5=off  GPIO_BIT5_Toggle=off  GPIO_Bit6=off  GPIO_BIT6_Toggle=off  GPIO_Bit7=off  GPIO_BIT7_Toggle=off
      settings: SourceProductName=Embedded Coder Support Package for Texas Instruments C2000 Processors  SourceProductBaseCode=TIC2000
  wires:
  Data Store Read/1 -> Digital Output/1
  Data Store Read1/1 -> Digital Output1/1

== system TEST_IPM_2_0/INT/AD2S1210 Init/Function-Call Subsystem4 ==
  function : TriggerPort  TriggerType=function-call  VariantControl=Variant
  Data Store Read : DataStoreRead  DataStoreName=ResloverA0
  Data Store Read1 : DataStoreRead  DataStoreName=ResloverA1
  Data Store Read2 : DataStoreRead  DataStoreName=ResloverWR
  Digital Output : c2837xDlib/Digital Output  GPIO_Number=GPIO56~GPIO63  GPIO_Bit0=off  GPIO_BIT0_Toggle=off  GPIO_Bit1=off  GPIO_BIT1_Toggle=off  GPIO_Bit2=on  GPIO_BIT2_Toggle=off  GPIO_Bit3=off  GPIO_BIT3_Toggle=off  GPIO_Bit4=off  GPIO_BIT4_Toggle=off  GPIO_Bit5=off  GPIO_BIT5_Toggle=off  GPIO_Bit6=off  GPIO_BIT6_Toggle=off  GPIO_Bit7=off  GPIO_BIT7_Toggle=off
      settings: SourceProductName=Embedded Coder Support Package for Texas Instruments C2000 Processors  SourceProductBaseCode=TIC2000
  Digital Output1 : c2837xDlib/Digital Output  GPIO_Number=GPIO56~GPIO63  GPIO_Bit0=off  GPIO_BIT0_Toggle=off  GPIO_Bit1=off  GPIO_BIT1_Toggle=off  GPIO_Bit2=off  GPIO_BIT2_Toggle=off  GPIO_Bit3=on  GPIO_BIT3_Toggle=off  GPIO_Bit4=off  GPIO_BIT4_Toggle=off  GPIO_Bit5=off  GPIO_BIT5_Toggle=off  GPIO_Bit6=off  GPIO_BIT6_Toggle=off  GPIO_Bit7=off  GPIO_BIT7_Toggle=off
      settings: SourceProductName=Embedded Coder Support Package for Texas Instruments C2000 Processors  SourceProductBaseCode=TIC2000
  Digital Output2 : c2837xDlib/Digital Output  GPIO_Number=GPIO48~GPIO55  GPIO_Bit0=off  GPIO_BIT0_Toggle=off  GPIO_Bit1=off  GPIO_BIT1_Toggle=off  GPIO_Bit2=off  GPIO_BIT2_Toggle=off  GPIO_Bit3=off  GPIO_BIT3_Toggle=off  GPIO_Bit4=off  GPIO_BIT4_Toggle=off  GPIO_Bit5=on  GPIO_BIT5_Toggle=off  GPIO_Bit6=off  GPIO_BIT6_Toggle=off  GPIO_Bit7=off  GPIO_BIT7_Toggle=off
      settings: SourceProductName=Embedded Coder Support Package for Texas Instruments C2000 Processors  SourceProductBaseCode=TIC2000
  wires:
  Data Store Read1/1 -> Digital Output1/1
  Data Store Read/1 -> Digital Output/1
  Data Store Read2/1 -> Digital Output2/1

== system TEST_IPM_2_0/INT/Data Buffer/Function-Call Subsystem ==
  function : TriggerPort  TriggerType=function-call  VariantControl=Variant
  Data Store Read : DataStoreRead  DataStoreName=DEKF_FLAG
  Data Store Read55 : DataStoreRead  DataStoreName=INITV_RS
  Data Store Read56 : DataStoreRead  DataStoreName=INITV_NDD
  Data Store Read57 : DataStoreRead  DataStoreName=INITV_NDQ
  Data Store Read58 : DataStoreRead  DataStoreName=INITV_NQQ
  Data Store Read59 : DataStoreRead  DataStoreName=INITV_PSI
  Data Store Read60 : DataStoreRead  DataStoreName=Id_FBK
  Data Store Read61 : DataStoreRead  DataStoreName=Iq_FBK
  Data Store Read62 : DataStoreRead  DataStoreName=UDOUT_Comp
  Data Store Read63 : DataStoreRead  DataStoreName=UQOUT_Comp
  Data Store Read64 : DataStoreRead  DataStoreName=N_FBK
  Data Store Read65 : DataStoreRead  DataStoreName=DEKF_Gamma
  Data Store Read66 : DataStoreRead  DataStoreName=DEKF_ComP
  Data Store Read68 : DataStoreRead  DataStoreName=DEKF_R
  Data Store Read69 : DataStoreRead  DataStoreName=DEKF_Qx
  Data Store Read70 : DataStoreRead  DataStoreName=DEKF_QpRs
  Data Store Read71 : DataStoreRead  DataStoreName=DEKF_QpLdd
  Data Store Read72 : DataStoreRead  DataStoreName=DEKF_QpLdq
  Data Store Read73 : DataStoreRead  DataStoreName=DEKF_QpLqq
  Data Store Read74 : DataStoreRead  DataStoreName=DEKF_QpPsi
  Data Store Read75 : DataStoreRead  DataStoreName=DEKF_Clear
  Data Type Conversion : DataTypeConversion  OutDataTypeStr=single
  Data Type Conversion1 : DataTypeConversion  OutDataTypeStr=single
  IPC Transmit : c2837xDlib/IPC Transmit  SelectChannel=0  EnableBlocking=off
      settings: SourceProductName=Embedded Coder Support Package for Texas Instruments C2000 Processors  SourceProductBaseCode=TIC2000
  LP_400Hz{,1..3} (4 alike) : dsparch4/Biquad Filter  Tag=BlockMethodSubSystem  FilterSource=Dialog parameters  CoeffSource=Specify via dialog  FilterObject=BQF  IIRFiltStruct=Direct form II  BiQuadCoeffs=[1 2 1 1 -1.76882785992372193 0.826201332947616107;1 2 1 1 -1.57523997778815161 0.626334259159141316]  ScaleValues=[0.014343368255973583;0.0127735703427474551;1]  IC=0  ICnum=0  ICden=0  a0Flag=Warning  optimizeScaleValues=on  ScaleValueMode=Specify via input port (g)  InputProcessing=Columns as channels (frame based)  roundingMode=Floor  overflowMode=off  scaleValueFracLength=14  denProdOutputFracLength=30  denAccumFracLength=30  secondMemoryFracLength=15
      settings: SourceProductName=DSP System Toolbox
  Mux : Mux  Inputs=22
  wires:
  Mux/1 -> IPC Transmit/1
  Data Store Read60/1 -> LP_400Hz/1
  Data Store Read61/1 -> LP_400Hz1/1
  Data Store Read62/1 -> LP_400Hz2/1
  Data Store Read63/1 -> LP_400Hz3/1
  Data Store Read64/1 -> Mux/5
  Data Store Read65/1 -> Mux/6
  Data Store Read66/1 -> Mux/7
  ? -> Mux/8
  Data Store Read68/1 -> Mux/9
  Data Store Read69/1 -> Mux/10
  Data Store Read70/1 -> Mux/11
  Data Store Read71/1 -> Mux/12
  Data Store Read72/1 -> Mux/13
  Data Store Read73/1 -> Mux/14
  Data Store Read74/1 -> Mux/15
  Data Store Read75/1 -> Data Type Conversion1/1
  Data Store Read55/1 -> Mux/17
  Data Store Read56/1 -> Mux/18
  Data Store Read57/1 -> Mux/19
  Data Store Read58/1 -> Mux/20
  Data Store Read59/1 -> Mux/21
  Data Store Read/1 -> Data Type Conversion/1
  Data Type Conversion/1 -> Mux/22
  Data Type Conversion1/1 -> Mux/16
  LP_400Hz/1 -> Mux/1
  LP_400Hz1/1 -> Mux/2
  LP_400Hz2/1 -> Mux/3
  LP_400Hz3/1 -> Mux/4

== system TEST_IPM_2_0/INT/Data Buffer/Function-Call Subsystem1 ==
  function : TriggerPort  TriggerType=function-call  VariantControl=Variant
  Data Store Write : DataStoreWrite  DataStoreName=iqObOUT
  Data Store Write1 : DataStoreWrite  DataStoreName=idObOUT
  Data Store Write27 : DataStoreWrite  DataStoreName=DEKF_LdEst
  Data Store Write28 : DataStoreWrite  DataStoreName=DEKF_LqEst
  Data Store Write29 : DataStoreWrite  DataStoreName=DEKF_PsiEst
  Data Store Write30 : DataStoreWrite  DataStoreName=DEKF_Rs
  Demux : Demux  Outputs=6
  IPC Receive : c2837xDlib/IPC Receive  SelectChannel=1  DataType=single  DataLength=6  EnableBlocking=off  SampleTime=-1
      settings: SourceProductName=Embedded Coder Support Package for Texas Instruments C2000 Processors  SourceProductBaseCode=TIC2000
  Terminator : Terminator
  wires:
  IPC Receive/1 -> Demux/1
  IPC Receive/2 -> Terminator/1
  Demux/1 -> Data Store Write30/1
  Demux/2 -> Data Store Write27/1
  Demux/3 -> Data Store Write28/1
  Demux/4 -> Data Store Write29/1
  Demux/5 -> Data Store Write1/1
  Demux/6 -> Data Store Write/1

== system TEST_IPM_2_0/INT/Data Buffer/Subsystem ==
  function : TriggerPort  TriggerType=function-call  VariantControl=Variant
  Data Store Read10 : DataStoreRead  DataStoreName=DEKF_Uqh
  Data Store Read11 : DataStoreRead  DataStoreName=N_400Hz
  Data Store Read12 : DataStoreRead  DataStoreName=N_NOFILTER
  Data Store Read6 : DataStoreRead  DataStoreName=ControlAng
  Data Store Read7 : DataStoreRead  DataStoreName=DEKF_Idh
  Data Store Read8 : DataStoreRead  DataStoreName=DEKF_Iqh
  Data Store Read9 : DataStoreRead  DataStoreName=DEKF_Udh
  MATLAB Function : MATLAB Function  TreatAsAtomicUnit=on
  wires:
  Data Store Read8/1 -> MATLAB Function/5(IqFBK)
  Data Store Read10/1 -> MATLAB Function/6(UqComP)
  Data Store Read9/1 -> MATLAB Function/3(UdComP)
  Data Store Read11/1 -> MATLAB Function/4(IqREF)
  Data Store Read6/1 -> MATLAB Function/7(Theta)
  Data Store Read7/1 -> MATLAB Function/2(IdFBK)
  Data Store Read12/1 -> MATLAB Function/1(IdREF)

== system TEST_IPM_2_0/INT/Extra Observer/Park Transformation2 ==
  Alpha : Inport
  Beta : Inport  Port=2
  theta : Inport  Port=3
  Add : Sum
  Add1 : Sum  Inputs=+-
  Gain : Gain  Gain=2*pi
  Product{,1..3} (4 alike) : Product
  Sin : Trigonometry  OutputSignalType=real
  Sin1 : Trigonometry  Operator=cos  OutputSignalType=real
  D : Outport
  Q : Outport  Port=2
  wires:
  Product/1 -> Add/1
  Sin/1 -> Product3/2, Product1/2
  Product1/1 -> Add/2
  Add1/1 -> Q/1
  Sin1/1 -> Product2/2, Product/2
  Product2/1 -> Add1/1
  Alpha/1 -> Product3/1, Product/1
  Beta/1 -> Product2/1, Product1/1
  Product3/1 -> Add1/2
  Add/1 -> D/1
  theta/1 -> Gain/1
  Gain/1 -> Sin/1, Sin1/1

== system TEST_IPM_2_0/INT/Extra Observer/Park Transformation3 ==
  Alpha : Inport
  Beta : Inport  Port=2
  theta : Inport  Port=3
  Add : Sum
  Add1 : Sum  Inputs=+-
  Gain : Gain  Gain=2*pi
  Product{,1..3} (4 alike) : Product
  Sin : Trigonometry  OutputSignalType=real
  Sin1 : Trigonometry  Operator=cos  OutputSignalType=real
  D : Outport
  Q : Outport  Port=2
  wires:
  Gain/1 -> Sin1/1, Sin/1
  theta/1 -> Gain/1
  Add/1 -> D/1
  Product3/1 -> Add1/2
  Beta/1 -> Product1/1, Product2/1
  Alpha/1 -> Product/1, Product3/1
  Product2/1 -> Add1/1
  Sin1/1 -> Product/2, Product2/2
  Add1/1 -> Q/1
  Product1/1 -> Add/2
  Sin/1 -> Product1/2, Product3/2
  Product/1 -> Add/1

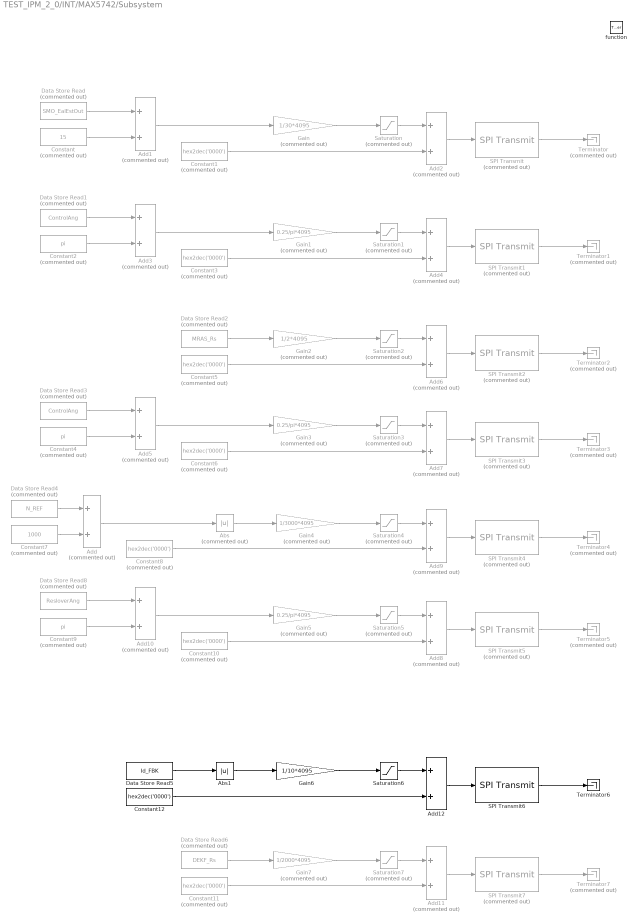
== system TEST_IPM_2_0/INT/MAX5742/Subsystem ==
  function : TriggerPort  TriggerType=function-call  VariantControl=Variant
  Abs : Abs  Commented=on
  Abs1 : Abs
  Add{,1..11} (12 alike) : Sum  Commented=on
  Add12 : Sum
  Constant : Constant  Commented=on  Value=15  OutDataTypeStr=single  SampleTime=-1
  Constant{1,3,5..6,8,10..11} (7 alike) : Constant  Commented=on  Value=hex2dec('0000')  OutDataTypeStr=uint16  SampleTime=-1
  Constant12 : Constant  Value=hex2dec('0000')  OutDataTypeStr=uint16  SampleTime=-1
  Constant2 : Constant  Commented=on  Value=pi  OutDataTypeStr=single  SampleTime=-1
  Constant4 : Constant  Commented=on  Value=pi  OutDataTypeStr=single  SampleTime=-1
  Constant7 : Constant  Commented=on  Value=1000  OutDataTypeStr=single  SampleTime=-1
  Constant9 : Constant  Commented=on  Value=pi  OutDataTypeStr=single  SampleTime=-1
  Data Store Read : DataStoreRead  Commented=on  DataStoreName=SMO_EalEstOut
  Data Store Read1 : DataStoreRead  Commented=on  DataStoreName=ControlAng
  Data Store Read2 : DataStoreRead  Commented=on  DataStoreName=MRAS_Rs
  Data Store Read3 : DataStoreRead  Commented=on  DataStoreName=ControlAng
  Data Store Read4 : DataStoreRead  Commented=on  DataStoreName=N_REF
  Data Store Read5 : DataStoreRead  DataStoreName=Id_FBK
  Data Store Read6 : DataStoreRead  Commented=on  DataStoreName=DEKF_Rs
  Data Store Read8 : DataStoreRead  Commented=on  DataStoreName=ResloverAng
  Gain : Gain  Commented=on  Gain=1/30*4095
  Gain1 : Gain  Commented=on  Gain=0.25/pi*4095
  Gain2 : Gain  Commented=on  Gain=1/2*4095
  Gain3 : Gain  Commented=on  Gain=0.25/pi*4095
  Gain4 : Gain  Commented=on  Gain=1/3000*4095
  Gain5 : Gain  Commented=on  Gain=0.25/pi*4095
  Gain6 : Gain  Gain=1/10*4095
  Gain7 : Gain  Commented=on  Gain=1/2000*4095
  SPI Transmit{,1..5,7} (7 alike) : c280xlib/SPI Transmit  Commented=on  SPISelect=SPI_B  ClockPolarity=Rising_edge  ClockPhase=No_delay  SPIModule=uint32(0)  Mode=Master  BusSpeed=uint32(1000000)  FirstBitToTransfer=Most significant bit (MSB)  ClockMode=0  BlockFunction=Write  EnableRegisterAddress=on  RegisterAddress=0  OutputDataType=int8  OutputDataLength=1  BlockingMode=off  DataBits=16  UseCustomSSPin=Provided by the SPI peripheral  ActiveLowSSPin=Active low  Pin=0
      settings: SourceProductName=Embedded Coder Support Package for Texas Instruments C2000 Processors  SourceProductBaseCode=TIC2000
  SPI Transmit6 : c280xlib/SPI Transmit  SPISelect=SPI_B  ClockPolarity=Rising_edge  ClockPhase=No_delay  SPIModule=uint32(0)  Mode=Master  BusSpeed=uint32(1000000)  FirstBitToTransfer=Most significant bit (MSB)  ClockMode=0  BlockFunction=Write  EnableRegisterAddress=on  RegisterAddress=0  OutputDataType=int8  OutputDataLength=1  BlockingMode=off  DataBits=16  UseCustomSSPin=Provided by the SPI peripheral  ActiveLowSSPin=Active low  Pin=0
      settings: SourceProductName=Embedded Coder Support Package for Texas Instruments C2000 Processors  SourceProductBaseCode=TIC2000
  Saturation{,1..5,7} (7 alike) : Saturate  Commented=on  UpperLimit=4095  LowerLimit=0  OutDataTypeStr=uint16
  Saturation6 : Saturate  UpperLimit=4095  LowerLimit=0  OutDataTypeStr=uint16
  Terminator{,1..5,7} (7 alike) : Terminator  Commented=on
  Terminator6 : Terminator
  wires:
  Constant1/1 -> Add2/2
  SPI Transmit/1 -> Terminator/1
  Saturation/1 -> Add2/1
  Add2/1 -> SPI Transmit/1
  Gain/1 -> Saturation/1
  Add1/1 -> Gain/1
  Data Store Read/1 -> Add1/1
  Constant/1 -> Add1/2
  Gain1/1 -> Saturation1/1
  Saturation1/1 -> Add4/1
  SPI Transmit1/1 -> Terminator1/1
  Constant3/1 -> Add4/2
  Add4/1 -> SPI Transmit1/1
  Add3/1 -> Gain1/1
  Constant2/1 -> Add3/2
  Data Store Read1/1 -> Add3/1
  Constant5/1 -> Add6/2
  Saturation2/1 -> Add6/1
  SPI Transmit2/1 -> Terminator2/1
  Gain2/1 -> Saturation2/1
  Add6/1 -> SPI Transmit2/1
  Data Store Read2/1 -> Gain2/1
  Gain3/1 -> Saturation3/1
  Saturation3/1 -> Add7/1
  Add7/1 -> SPI Transmit3/1
  Constant6/1 -> Add7/2
  Constant4/1 -> Add5/2
  Data Store Read3/1 -> Add5/1
  Add5/1 -> Gain3/1
  SPI Transmit3/1 -> Terminator3/1
  Saturation4/1 -> Add9/1
  Add9/1 -> SPI Transmit4/1
  SPI Transmit4/1 -> Terminator4/1
  Constant8/1 -> Add9/2
  Gain4/1 -> Saturation4/1
  Add/1 -> Abs/1
  Abs/1 -> Gain4/1
  Data Store Read4/1 -> Add/1
  Constant7/1 -> Add/2
  Constant9/1 -> Add10/2
  Data Store Read8/1 -> Add10/1
  Add10/1 -> Gain5/1
  SPI Transmit5/1 -> Terminator5/1
  Saturation5/1 -> Add8/1
  Gain5/1 -> Saturation5/1
  Add8/1 -> SPI Transmit5/1
  Constant10/1 -> Add8/2
  Add12/1 -> SPI Transmit6/1
  Data Store Read5/1 -> Abs1/1
  Abs1/1 -> Gain6/1
  Saturation6/1 -> Add12/1
  Constant12/1 -> Add12/2
  SPI Transmit6/1 -> Terminator6/1
  Gain6/1 -> Saturation6/1
  Gain7/1 -> Saturation7/1
  Data Store Read6/1 -> Gain7/1
  Add11/1 -> SPI Transmit7/1
  SPI Transmit7/1 -> Terminator7/1
  Constant11/1 -> Add11/2
  Saturation7/1 -> Add11/1
